simulink model "generic_mcycle"  (Simulink 10.3)
settings: Solver=ode45  StartTime=0.0  StopTime=inf  RelTol=1e-3  EnableMultiTasking=on
libraries: MCycleMaker4SL x1, simulink x1
settings Model: Creator=IPG  LastModifiedBy=IPG  MultithreadedSim=on  ExtModeAutoUpdateStatusClock=off
settings DataIOCC: LimitDataPoints=on  SignalLoggingName=sigsOut
settings OptimizationCC: BooleanDataType=off  InitFltsAndDblsToZero=on
settings DebuggingCC: SaveWithParameterizedLinksMsg=none  SignalResolutionControl=TryResolveAllWithWarning  MultiTaskDSMMsg=warning  MultiTaskCondExecSysMsg=none  SFExecutionAtInitializationDiag=warning
settings HardwareCC: TargetUnknown=on
settings CodeAppCC: MaxIdLength=63
settings GRTTargetCC: TargetFcnLib=ansi_tfl_tmw.mat

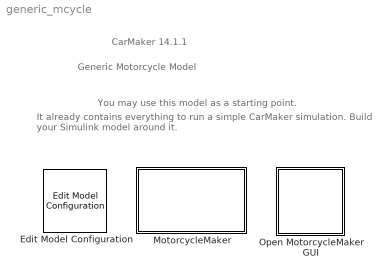
== system generic_mcycle ==
  note: Generic Motorcycle Model
  note: CarMaker 14.1.1
  note: You may use this model as a starting point.
  note: It already contains everything to run a simple CarMaker simulation.
      | Build your Simulink model around it.
  Edit Model Configuration : MCycleMaker4SL/Edit Model Configuration  SFunctionModules=''
  MotorcycleMaker : Subsystem  TreatAsAtomicUnit=on
      mask Display: image(imread('MCycleMakerSys.png'));
  Open MotorcycleMaker GUI : Subsystem  LoadFcn=if ~length(which('cmself')), cmenv; end
      settings: OpenFcn=cmblockmagic('gui_fix_display'); MM_Simulink
      mask Display: image(imread('MCycleMakerGUI.png'));

== system generic_mcycle/MotorcycleMaker ==
  CM_FIRST : Subsystem
  CM_LAST : Subsystem
  DrivMan : Subsystem
  Ground : Ground
  Terminator : Terminator
  Vehicle : Subsystem  TreatAsAtomicUnit=on
  VehicleControl : Subsystem
  wires:
  CM_FIRST/2(Env.Misc) -> DrivMan/2(Env.Misc)
  VehicleControl/2(Vhcl.Model.Source) -> Vehicle/2(Vhcl.Model.Source)
  VehicleControl/7(VhclCtrl.PT) -> Vehicle/7(VhclCtrl.PT)
  VehicleControl/6(VhclCtrl.Brake) -> Vehicle/6(VhclCtrl.Brake)
  VehicleControl/5(Vhcl.Misc) -> Vehicle/5(Vhcl.Misc)
  VehicleControl/4(Vhcl.Wheel.In) -> Vehicle/4(Vhcl.Wheel.In)
  VehicleControl/3(VhclCtrl.Steering) -> Vehicle/3(VhclCtrl.Steering)
  VehicleControl/1(Sync_Out) -> Vehicle/1(Sync_In)
  Vehicle/1(Sync_Out) -> CM_LAST/1(Sync_In)
  Ground/1 -> CM_FIRST/1(Sync_In)
  CM_LAST/1(Sync_Out) -> Terminator/1
  CM_FIRST/1(Sync_Out) -> DrivMan/1(Sync_In)
  DrivMan/1(Sync_Out) -> VehicleControl/1(Sync_In)
  DrivMan/2(DrivMan.Out) -> VehicleControl/2(DrivMan.In)

== system generic_mcycle/Open MotorcycleMaker GUI ==
  S-Function : S-Function  FunctionName=cm_gui  SFunctionDeploymentMode=off  EnableBusSupport=off

== system generic_mcycle/MotorcycleMaker/CM_FIRST ==
  Sync_In : Inport
  BusCreator1 : BusCreator  Inputs=8
  BusCreator2 : BusCreator  Inputs=6
  Demux1 : Demux  Outputs=14
      settings: DisplayOption=none
  Environment : S-Function  FunctionName=MM_Sfun  Parameters='Environment'  SFunctionDeploymentMode=off  EnableBusSupport=off
  IoIn : S-Function  FunctionName=MM_Sfun  Parameters='IoIn'  SFunctionDeploymentMode=off  EnableBusSupport=off
  Terminator : Terminator
  Sync_Out : Outport  VectorParamsAs1DForOutWhenUnconnected=off
  Env.Misc : Outport  Port=2  VectorParamsAs1DForOutWhenUnconnected=off
  wires:
  BusCreator2/1 -> Terminator/1  "IF Environment (in)"
  BusCreator1/1 -> Env.Misc/1
  Demux1/14 -> BusCreator2/6  "Env sRoad"
  Demux1/13 -> BusCreator2/5  "Env PoI_GCS Elev"
  Demux1/12 -> BusCreator2/4  "Env PoI_GCS Lat"
  Demux1/11 -> BusCreator2/3  "Env PoI_GCS Long"
  Demux1/10 -> BusCreator2/2  "Env Time"
  Demux1/9 -> BusCreator2/1  "Env yDay"
  Demux1/8 -> BusCreator1/8  "Env WindVel_tot z"
  Demux1/7 -> BusCreator1/7  "Env WindVel_tot y"
  Demux1/6 -> BusCreator1/6  "Env WindVel_tot x"
  Demux1/5 -> BusCreator1/5  "Env SolarRadiation"
  Demux1/4 -> BusCreator1/4  "Env AirHumidity"
  Demux1/3 -> BusCreator1/3  "Env AirPressure"
  Demux1/2 -> BusCreator1/2  "Env AirDensity"
  Demux1/1 -> BusCreator1/1  "Env Temperature"
  Sync_In/1 -> IoIn/1
  IoIn/1 -> Environment/1
  Environment/1 -> Sync_Out/1
  Environment/2 -> Demux1/1

== system generic_mcycle/MotorcycleMaker/CM_LAST ==
  Sync_In : Inport
  CM_User : S-Function  FunctionName=MM_Sfun  Parameters='CM_User'  SFunctionDeploymentMode=off  EnableBusSupport=off
  IoOut : S-Function  FunctionName=MM_Sfun  Parameters='IoOut'  SFunctionDeploymentMode=off  EnableBusSupport=off
  Sync_Out : Outport  VectorParamsAs1DForOutWhenUnconnected=off
  wires:
  IoOut/1 -> Sync_Out/1
  CM_User/1 -> IoOut/1
  Sync_In/1 -> CM_User/1

== system generic_mcycle/MotorcycleMaker/DrivMan ==
  note: There's rarely a reason to override DrivMan signals.
      | Use the VehicleControl interface for this purpose.
  Sync_In : Inport
  Env.Misc : Inport  Port=2
  BusCreator1 : BusCreator  Inputs=23
  Demux1 : Demux  Outputs=23
      settings: DisplayOption=none
  DrivMan : S-Function  FunctionName=MM_Sfun  Parameters='DrivMan'  SFunctionDeploymentMode=off  EnableBusSupport=off
  Sync_Out : Outport  VectorParamsAs1DForOutWhenUnconnected=off
  DrivMan.Out : Outport  Port=2  VectorParamsAs1DForOutWhenUnconnected=off
  wires:
  Demux1/8 -> BusCreator1/8  "DrivMan SelectorCtrl"
  Demux1/7 -> BusCreator1/7  "DrivMan UserSignal4"
  Demux1/6 -> BusCreator1/6  "DrivMan UserSignal3"
  Demux1/5 -> BusCreator1/5  "DrivMan UserSignal2"
  Demux1/4 -> BusCreator1/4  "DrivMan UserSignal1"
  Demux1/3 -> BusCreator1/3  "DrivMan UserSignal0"
  Demux1/2 -> BusCreator1/2  "DrivMan Key"
  Demux1/1 -> BusCreator1/1  "DrivMan SST"
  DrivMan/1 -> Sync_Out/1
  Sync_In/1 -> DrivMan/1
  Env.Misc/1 -> DrivMan/2
  DrivMan/2 -> Demux1/1
  BusCreator1/1 -> DrivMan.Out/1
  Demux1/9 -> BusCreator1/9  "DrivMan DigitalSelectorCtrl0"
  Demux1/10 -> BusCreator1/10  "DrivMan DigitalSelectorCtrl1"
  Demux1/11 -> BusCreator1/11  "DrivMan DigitalSelectorCtrl2"
  Demux1/23 -> BusCreator1/23  "DrivMan Rider RollAngVel"
  Demux1/22 -> BusCreator1/22  "DrivMan Rider RollAng"
  Demux1/21 -> BusCreator1/21  "DrivMan Steering Trq"
  Demux1/20 -> BusCreator1/20  "DrivMan Steering AngAcc"
  Demux1/19 -> BusCreator1/19  "DrivMan Steering AngVel"
  Demux1/18 -> BusCreator1/18  "DrivMan Steering Ang"
  Demux1/17 -> BusCreator1/17  "DrivMan Gas"
  Demux1/16 -> BusCreator1/16  "DrivMan Clutch"
  Demux1/15 -> BusCreator1/15  "DrivMan BrakePark"
  Demux1/14 -> BusCreator1/14  "DrivMan BrakeLever"
  Demux1/13 -> BusCreator1/13  "DrivMan Brake"
  Demux1/12 -> BusCreator1/12  "DrivMan GearNo"

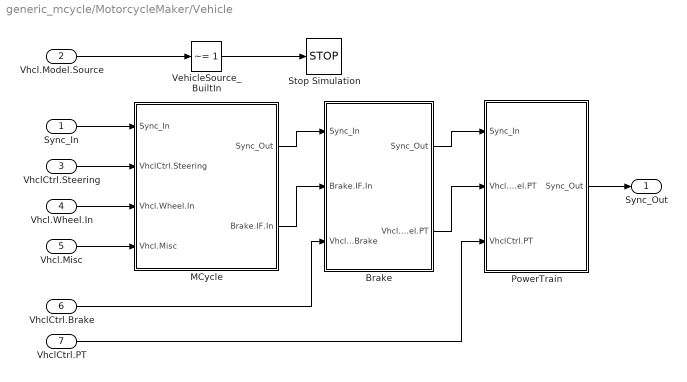
== system generic_mcycle/MotorcycleMaker/Vehicle ==
  Sync_In : Inport
  Vhcl.Model.Source : Inport  Port=2
  VhclCtrl.Steering : Inport  Port=3
  Vhcl.Wheel.In : Inport  Port=4
  Vhcl.Misc : Inport  Port=5
  VhclCtrl.Brake : Inport  Port=6
  VhclCtrl.PT : Inport  Port=7
  Brake : Subsystem
  MCycle : Subsystem
  PowerTrain : Subsystem
  Stop Simulation : Stop
  VehicleSource_BuiltIn : simulink/Logic and Bit Operations/Compare To Constant  relop=~=  const=1  OutDataTypeStr=boolean  ZeroCross=off
  Sync_Out : Outport  VectorParamsAs1DForOutWhenUnconnected=off
  wires:
  Vhcl.Model.Source/1 -> VehicleSource_BuiltIn/1
  Sync_In/1 -> MCycle/1(Sync_In)
  VhclCtrl.Steering/1 -> MCycle/2(VhclCtrl.Steering)
  Vhcl.Wheel.In/1 -> MCycle/3(Vhcl.Wheel.In)
  Vhcl.Misc/1 -> MCycle/4(Vhcl.Misc)
  PowerTrain/1(Sync_Out) -> Sync_Out/1
  VhclCtrl.Brake/1 -> Brake/3(VhclCtrl.Brake)
  MCycle/2(Brake.IF.In) -> Brake/2(Brake.IF.In)
  MCycle/1(Sync_Out) -> Brake/1(Sync_In)
  Brake/1(Sync_Out) -> PowerTrain/1(Sync_In)
  VhclCtrl.PT/1 -> PowerTrain/3(VhclCtrl.PT)
  VehicleSource_BuiltIn/1 -> Stop Simulation/1
  Brake/2(Vhcl.Wheel.PT) -> PowerTrain/2(Vhcl.Wheel.PT)

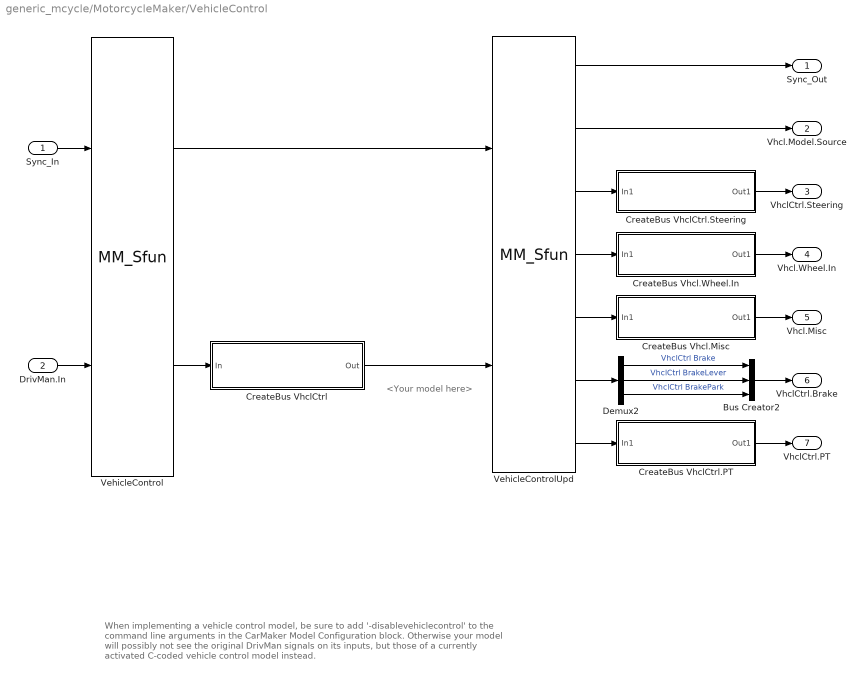
== system generic_mcycle/MotorcycleMaker/VehicleControl ==
  note: When implementing a vehicle control model,
      | be sure to add '-disablevehiclecontrol' to the command line arguments
      | in the CarMaker Model Configuration block.
      | Otherwise your model will possibly not see the original DrivMan signals
      | on its inputs, but those of a currently activated C-coded vehicle control model instead.
  note: <Your model here>
  Sync_In : Inport
  DrivMan.In : Inport  Port=2
  Bus Creator2 : BusCreator  Inputs=3
  CreateBus Vhcl.Misc : Subsystem
  CreateBus Vhcl.Wheel.In : Subsystem
  CreateBus VhclCtrl : Subsystem
  CreateBus VhclCtrl.PT : Subsystem
  CreateBus VhclCtrl.Steering : Subsystem
  Demux2 : Demux  Outputs=3
      settings: DisplayOption=none
  VehicleControl : S-Function  FunctionName=MM_Sfun  Parameters='VehicleControl'  SFunctionDeploymentMode=off  EnableBusSupport=off
  VehicleControlUpd : S-Function  FunctionName=MM_Sfun  Parameters='VehicleControlUpd'  SFunctionDeploymentMode=off  EnableBusSupport=off
  Sync_Out : Outport  VectorParamsAs1DForOutWhenUnconnected=off
  Vhcl.Model.Source : Outport  Port=2  VectorParamsAs1DForOutWhenUnconnected=off
  VhclCtrl.Steering : Outport  Port=3  VectorParamsAs1DForOutWhenUnconnected=off
  Vhcl.Wheel.In : Outport  Port=4  VectorParamsAs1DForOutWhenUnconnected=off
  Vhcl.Misc : Outport  Port=5  VectorParamsAs1DForOutWhenUnconnected=off
  VhclCtrl.Brake : Outport  Port=6  VectorParamsAs1DForOutWhenUnconnected=off
  VhclCtrl.PT : Outport  Port=7  VectorParamsAs1DForOutWhenUnconnected=off
  wires:
  Demux2/1 -> Bus Creator2/1  "VhclCtrl Brake"
  Demux2/2 -> Bus Creator2/2  "VhclCtrl BrakeLever"
  VehicleControlUpd/1 -> Sync_Out/1
  CreateBus VhclCtrl.Steering/1(Out1) -> VhclCtrl.Steering/1
  Bus Creator2/1 -> VhclCtrl.Brake/1
  CreateBus VhclCtrl.PT/1(Out1) -> VhclCtrl.PT/1
  Sync_In/1 -> VehicleControl/1
  VehicleControl/1 -> VehicleControlUpd/1
  DrivMan.In/1 -> VehicleControl/2
  CreateBus Vhcl.Wheel.In/1(Out1) -> Vhcl.Wheel.In/1
  CreateBus Vhcl.Misc/1(Out1) -> Vhcl.Misc/1
  VehicleControlUpd/3 -> CreateBus VhclCtrl.Steering/1(In1)
  VehicleControlUpd/7 -> CreateBus VhclCtrl.PT/1(In1)
  VehicleControlUpd/6 -> Demux2/1
  VehicleControlUpd/5 -> CreateBus Vhcl.Misc/1(In1)
  VehicleControlUpd/4 -> CreateBus Vhcl.Wheel.In/1(In1)
  VehicleControlUpd/2 -> Vhcl.Model.Source/1
  Demux2/3 -> Bus Creator2/3  "VhclCtrl BrakePark"
  VehicleControl/2 -> CreateBus VhclCtrl/1(In)
  CreateBus VhclCtrl/1(Out) -> VehicleControlUpd/2

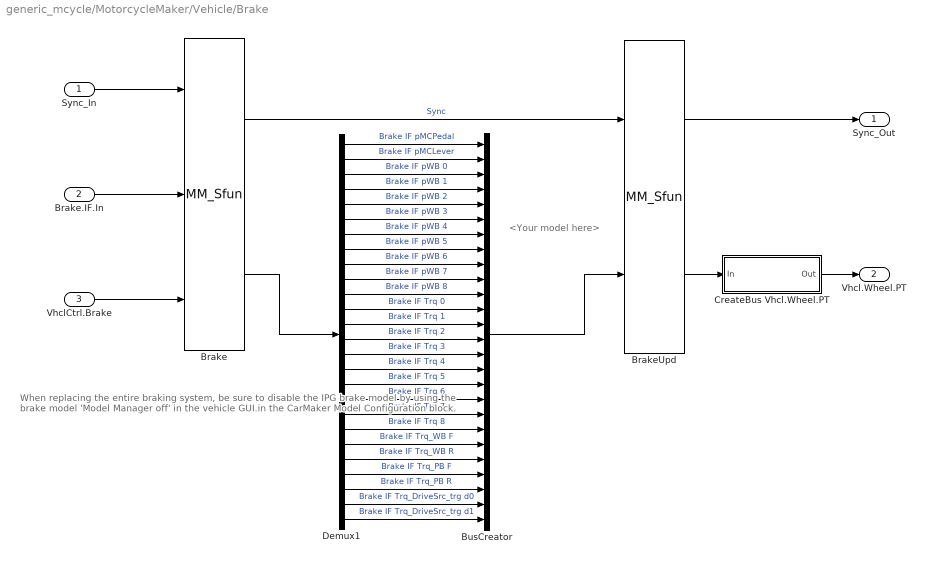
== system generic_mcycle/MotorcycleMaker/Vehicle/Brake ==
  note: When replacing the entire braking system,
      | be sure to disable the IPG brake model by using the brake
      | model 'Model Manager off' in the vehicle GUI.in the CarMaker Model Configuration block.
  note: <Your model here>
  Sync_In : Inport
  Brake.IF.In : Inport  Port=2
  VhclCtrl.Brake : Inport  Port=3
  Brake : S-Function  FunctionName=MM_Sfun  Parameters='Brake'  SFunctionDeploymentMode=off  EnableBusSupport=off
  BrakeUpd : S-Function  FunctionName=MM_Sfun  Parameters='BrakeUpd'  SFunctionDeploymentMode=off  EnableBusSupport=off
  BusCreator : BusCreator  Inputs=26
  CreateBus Vhcl.Wheel.PT : Subsystem
  Demux1 : Demux  Outputs=26
      settings: DisplayOption=none
  Sync_Out : Outport  VectorParamsAs1DForOutWhenUnconnected=off
  Vhcl.Wheel.PT : Outport  Port=2  VectorParamsAs1DForOutWhenUnconnected=off
  wires:
  Demux1/26 -> BusCreator/26  "Brake IF Trq_DriveSrc_trg d1"
  Demux1/25 -> BusCreator/25  "Brake IF Trq_DriveSrc_trg d0"
  Demux1/24 -> BusCreator/24  "Brake IF Trq_PB R"
  Demux1/23 -> BusCreator/23  "Brake IF Trq_PB F"
  Demux1/22 -> BusCreator/22  "Brake IF Trq_WB R"
  Demux1/21 -> BusCreator/21  "Brake IF Trq_WB F"
  Demux1/20 -> BusCreator/20  "Brake IF Trq 8"
  Demux1/19 -> BusCreator/19  "Brake IF Trq 7"
  Demux1/18 -> BusCreator/18  "Brake IF Trq 6"
  Demux1/17 -> BusCreator/17  "Brake IF Trq 5"
  Demux1/16 -> BusCreator/16  "Brake IF Trq 4"
  Demux1/15 -> BusCreator/15  "Brake IF Trq 3"
  Demux1/14 -> BusCreator/14  "Brake IF Trq 2"
  Demux1/13 -> BusCreator/13  "Brake IF Trq 1"
  Demux1/12 -> BusCreator/12  "Brake IF Trq 0"
  Demux1/11 -> BusCreator/11  "Brake IF pWB 8"
  Demux1/10 -> BusCreator/10  "Brake IF pWB 7"
  Demux1/9 -> BusCreator/9  "Brake IF pWB 6"
  Demux1/8 -> BusCreator/8  "Brake IF pWB 5"
  Demux1/7 -> BusCreator/7  "Brake IF pWB 4"
  Demux1/6 -> BusCreator/6  "Brake IF pWB 3"
  Demux1/5 -> BusCreator/5  "Brake IF pWB 2"
  Demux1/4 -> BusCreator/4  "Brake IF pWB 1"
  Demux1/3 -> BusCreator/3  "Brake IF pWB 0"
  Demux1/2 -> BusCreator/2  "Brake IF pMCLever"
  Demux1/1 -> BusCreator/1  "Brake IF pMCPedal"
  Sync_In/1 -> Brake/1
  VhclCtrl.Brake/1 -> Brake/3
  Brake.IF.In/1 -> Brake/2
  Brake/1 -> BrakeUpd/1  "Sync"
  BrakeUpd/1 -> Sync_Out/1
  Brake/2 -> Demux1/1
  BusCreator/1 -> BrakeUpd/2
  BrakeUpd/2 -> CreateBus Vhcl.Wheel.PT/1(In)
  CreateBus Vhcl.Wheel.PT/1(Out) -> Vhcl.Wheel.PT/1

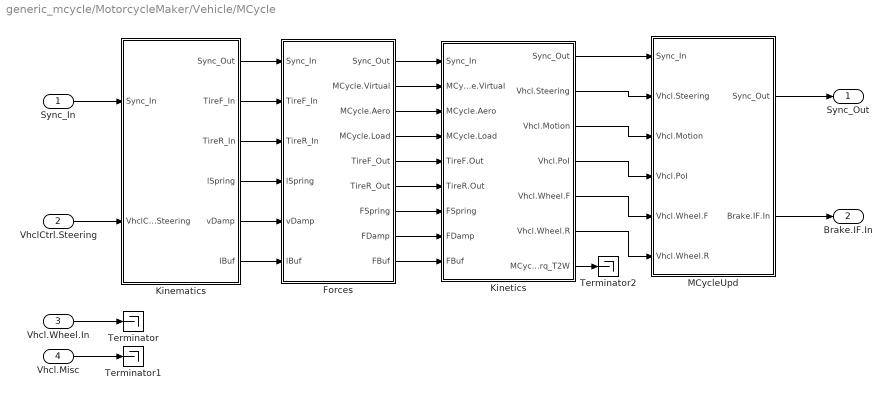
== system generic_mcycle/MotorcycleMaker/Vehicle/MCycle ==
  Sync_In : Inport
  VhclCtrl.Steering : Inport  Port=2
  Vhcl.Wheel.In : Inport  Port=3
  Vhcl.Misc : Inport  Port=4
  Forces : Subsystem
  Kinematics : Subsystem
  Kinetics : Subsystem
  MCycleUpd : Subsystem
  Terminator : Terminator
  Terminator1 : Terminator
  Terminator2 : Terminator
  Sync_Out : Outport  VectorParamsAs1DForOutWhenUnconnected=off
  Brake.IF.In : Outport  Port=2  VectorParamsAs1DForOutWhenUnconnected=off
  wires:
  Vhcl.Wheel.In/1 -> Terminator/1
  Vhcl.Misc/1 -> Terminator1/1
  MCycleUpd/1(Sync_Out) -> Sync_Out/1
  MCycleUpd/2(Brake.IF.In) -> Brake.IF.In/1
  Kinetics/1(Sync_Out) -> MCycleUpd/1(Sync_In)
  Kinetics/2(Vhcl.Steering) -> MCycleUpd/2(Vhcl.Steering)
  Kinetics/3(Vhcl.Motion) -> MCycleUpd/3(Vhcl.Motion)
  Kinetics/4(Vhcl.PoI) -> MCycleUpd/4(Vhcl.PoI)
  Kinetics/5(Vhcl.Wheel.F) -> MCycleUpd/5(Vhcl.Wheel.F)
  Kinetics/6(Vhcl.Wheel.R) -> MCycleUpd/6(Vhcl.Wheel.R)
  Sync_In/1 -> Kinematics/1(Sync_In)
  VhclCtrl.Steering/1 -> Kinematics/2(VhclCtrl.Steering)
  Kinematics/1(Sync_Out) -> Forces/1(Sync_In)
  Kinematics/4(lSpring) -> Forces/4(lSpring)
  Kinematics/5(vDamp) -> Forces/5(vDamp)
  Forces/1(Sync_Out) -> Kinetics/1(Sync_In)
  Forces/2(MCycle.Virtual) -> Kinetics/2(MCycle.Virtual)
  Forces/3(MCycle.Aero) -> Kinetics/3(MCycle.Aero)
  Forces/4(MCycle.Load) -> Kinetics/4(MCycle.Load)
  Forces/7(FSpring) -> Kinetics/7(FSpring)
  Forces/8(FDamp) -> Kinetics/8(FDamp)
  Forces/5(TireF_Out) -> Kinetics/5(TireF.Out)
  Forces/6(TireR_Out) -> Kinetics/6(TireR.Out)
  Kinematics/2(TireF_In) -> Forces/2(TireF_In)
  Kinematics/3(TireR_In) -> Forces/3(TireR_In)
  Kinetics/7(MCycle.Trq_T2W) -> Terminator2/1
  Forces/9(FBuf) -> Kinetics/9(FBuf)
  Kinematics/6(lBuf) -> Forces/6(lBuf)

== system generic_mcycle/MotorcycleMaker/Vehicle/PowerTrain ==
  note: <Your model here>
  note: When replacing the entire powertrain,
      | be sure to disable the IPG powertrain model by using the powertrain
      | model 'Model Manager off' in the vehicle GUI.
  Sync_In : Inport
  Vhcl.Wheel.PT : Inport  Port=2
  VhclCtrl.PT : Inport  Port=3
  BusCreator : BusCreator  Inputs=23
  Demux : Demux  Outputs=23
      settings: DisplayOption=none
  PowerTrain : S-Function  FunctionName=MM_Sfun  Parameters='PowerTrain'  SFunctionDeploymentMode=off  EnableBusSupport=off
  PowerTrainUpd : S-Function  FunctionName=MM_Sfun  Parameters='PowerTrainUpd'  SFunctionDeploymentMode=off  EnableBusSupport=off
  Sync_Out : Outport  VectorParamsAs1DForOutWhenUnconnected=off
  wires:
  Demux/23 -> BusCreator/23  "PT IF WR Trq_BrakeReg_max"
  Demux/22 -> BusCreator/22  "PT IF WR Trq_BrakeReg"
  Demux/21 -> BusCreator/21  "PT IF WR Trq_Supp2WC"
  Demux/20 -> BusCreator/20  "PT IF WR Trq_Drive"
  Demux/19 -> BusCreator/19  "PT IF WR Trq_B2W"
  Demux/18 -> BusCreator/18  "PT IF WR rotv"
  Demux/17 -> BusCreator/17  "PT IF WR rot"
  Demux/16 -> BusCreator/16  "PT IF WF Trq_BrakeReg_max"
  Demux/15 -> BusCreator/15  "PT IF WF Trq_BrakeReg"
  Demux/14 -> BusCreator/14  "PT IF WF Trq_Supp2WC"
  Demux/13 -> BusCreator/13  "PT IF WF Trq_Drive"
  Demux/12 -> BusCreator/12  "PT IF WF Trq_B2W"
  Demux/11 -> BusCreator/11  "PT IF WF rotv"
  Demux/10 -> BusCreator/10  "PT IF WF rot"
  Demux/9 -> BusCreator/9  "PT IF DL_iDiff_mean"
  Demux/8 -> BusCreator/8  "PT IF Trq_Supp2Bdy1 z"
  Demux/7 -> BusCreator/7  "PT IF Trq_Supp2Bdy1 y"
  Demux/6 -> BusCreator/6  "PT IF Trq_Supp2Bdy1 x"
  Demux/5 -> BusCreator/5  "PT IF Engine_rotv"
  Demux/4 -> BusCreator/4  "PT IF GearNo"
  Demux/3 -> BusCreator/3  "PT IF OperationError"
  Demux/2 -> BusCreator/2  "PT IF OperationState"
  Demux/1 -> BusCreator/1  "PT IF Ignition"
  BusCreator/1 -> PowerTrainUpd/2
  PowerTrain/1 -> PowerTrainUpd/1  "Sync"
  PowerTrainUpd/1 -> Sync_Out/1
  Sync_In/1 -> PowerTrain/1
  PowerTrain/2 -> Demux/1
  VhclCtrl.PT/1 -> PowerTrain/3
  Vhcl.Wheel.PT/1 -> PowerTrain/2

== system generic_mcycle/MotorcycleMaker/VehicleControl/CreateBus Vhcl.Misc ==
  In1 : Inport
  BusCreator : BusCreator  Inputs=6
  Demux : Demux  Outputs=6
      settings: DisplayOption=none
  Out1 : Outport  VectorParamsAs1DForOutWhenUnconnected=off
  wires:
  Demux/6 -> BusCreator/6  "Vhcl Wind_vel_0 z"
  Demux/5 -> BusCreator/5  "Vhcl Wind_vel_0 y"
  Demux/4 -> BusCreator/4  "Vhcl Wind_vel_0 x"
  Demux/3 -> BusCreator/3  "Vhcl Trq_DL2Bdy1 z"
  Demux/2 -> BusCreator/2  "Vhcl Trq_DL2Bdy1 y"
  Demux/1 -> BusCreator/1  "Vhcl Trq_DL2Bdy1 x"
  BusCreator/1 -> Out1/1
  In1/1 -> Demux/1

== system generic_mcycle/MotorcycleMaker/VehicleControl/CreateBus Vhcl.Wheel.In ==
  In1 : Inport
  Bus Creator1 : BusCreator  Inputs=6
  Demux1 : Demux  Outputs=6
      settings: DisplayOption=none
  Out1 : Outport  VectorParamsAs1DForOutWhenUnconnected=off
  wires:
  In1/1 -> Demux1/1
  Bus Creator1/1 -> Out1/1
  Demux1/1 -> Bus Creator1/1  "Vhcl Wheel F Trq_B2WC"
  Demux1/2 -> Bus Creator1/2  "Vhcl Wheel F Trq_DL2WC"
  Demux1/3 -> Bus Creator1/3  "Vhcl Wheel F rotv"
  Demux1/4 -> Bus Creator1/4  "Vhcl Wheel R Trq_B2WC"
  Demux1/5 -> Bus Creator1/5  "Vhcl Wheel R Trq_DL2WC"
  Demux1/6 -> Bus Creator1/6  "Vhcl Wheel R rotv"

== system generic_mcycle/MotorcycleMaker/VehicleControl/CreateBus VhclCtrl ==
  In : Inport
  BusCreator : BusCreator  Inputs=32
  Demux : Demux  Outputs=32
      settings: DisplayOption=none
  Out : Outport  VectorParamsAs1DForOutWhenUnconnected=off
  wires:
  BusCreator/1 -> Out/1
  In/1 -> Demux/1
  Demux/1 -> BusCreator/1  "VhclCtrl SST"
  Demux/2 -> BusCreator/2  "VhclCtrl Key"
  Demux/3 -> BusCreator/3  "VhclCtrl UserSignal0"
  Demux/4 -> BusCreator/4  "VhclCtrl UserSignal1"
  Demux/5 -> BusCreator/5  "VhclCtrl UserSignal2"
  Demux/6 -> BusCreator/6  "VhclCtrl UserSignal3"
  Demux/7 -> BusCreator/7  "VhclCtrl UserSignal4"
  Demux/8 -> BusCreator/8  "VhclCtrl GearNo"
  Demux/9 -> BusCreator/9  "VhclCtrl SelectorCtrl"
  Demux/10 -> BusCreator/10  "VhclCtrl Brake"
  Demux/11 -> BusCreator/11  "VhclCtrl BrakeLever"
  Demux/12 -> BusCreator/12  "VhclCtrl BrakePark"
  Demux/13 -> BusCreator/13  "VhclCtrl Clutch"
  Demux/14 -> BusCreator/14  "VhclCtrl Gas"
  Demux/15 -> BusCreator/15  "VhclCtrl Steering Ang"
  Demux/16 -> BusCreator/16  "VhclCtrl Steering AngVel"
  Demux/17 -> BusCreator/17  "VhclCtrl Steering AngAcc"
  Demux/18 -> BusCreator/18  "VhclCtrl Steering Trq"
  Demux/19 -> BusCreator/19  "VhclCtrl Rider RollAng"
  Demux/20 -> BusCreator/20  "VhclCtrl Rider RollAngVel"
  Demux/21 -> BusCreator/21  "VhclCtrl Lights LowBeam"
  Demux/22 -> BusCreator/22  "VhclCtrl Lights HighBeam"
  Demux/23 -> BusCreator/23  "VhclCtrl Lights Daytime"
  Demux/24 -> BusCreator/24  "VhclCtrl Lights ParkL"
  Demux/25 -> BusCreator/25  "VhclCtrl Lights ParkR"
  Demux/26 -> BusCreator/26  "VhclCtrl Lights IndL"
  Demux/27 -> BusCreator/27  "VhclCtrl Lights IndR"
  Demux/28 -> BusCreator/28  "VhclCtrl Lights FogFrontL"
  Demux/29 -> BusCreator/29  "VhclCtrl Lights FogFrontR"
  Demux/30 -> BusCreator/30  "VhclCtrl Lights FogRear"
  Demux/31 -> BusCreator/31  "VhclCtrl Lights Brake"
  Demux/32 -> BusCreator/32  "VhclCtrl Lights Reverse"

== system generic_mcycle/MotorcycleMaker/VehicleControl/CreateBus VhclCtrl.PT ==
  In1 : Inport
  BusCreator : BusCreator  Inputs=12
  Demux : Demux  Outputs=12
      settings: DisplayOption=none
  Out1 : Outport  VectorParamsAs1DForOutWhenUnconnected=off
  wires:
  Demux/12 -> BusCreator/12  "VhclCtrl Brake"
  Demux/11 -> BusCreator/11  "VhclCtrl Gas"
  Demux/10 -> BusCreator/10  "VhclCtrl Clutch"
  Demux/9 -> BusCreator/9  "VhclCtrl SelectorCtrl"
  Demux/8 -> BusCreator/8  "VhclCtrl GearNo"
  Demux/7 -> BusCreator/7  "VhclCtrl UserSignal4"
  Demux/6 -> BusCreator/6  "VhclCtrl UserSignal3"
  Demux/5 -> BusCreator/5  "VhclCtrl UserSignal2"
  Demux/4 -> BusCreator/4  "VhclCtrl UserSignal1"
  Demux/3 -> BusCreator/3  "VhclCtrl UserSignal0"
  Demux/2 -> BusCreator/2  "VhclCtrl Key"
  Demux/1 -> BusCreator/1  "VhclCtrl SST"
  BusCreator/1 -> Out1/1
  In1/1 -> Demux/1

== system generic_mcycle/MotorcycleMaker/VehicleControl/CreateBus VhclCtrl.Steering ==
  In1 : Inport
  BusCreator : BusCreator  Inputs=5
  Demux : Demux  Outputs=5
      settings: DisplayOption=none
  Out1 : Outport  VectorParamsAs1DForOutWhenUnconnected=off
  wires:
  Demux/5 -> BusCreator/5  "VhclCtrl Steering SteerByTrq"
  Demux/4 -> BusCreator/4  "VhclCtrl Steering Trq"
  Demux/3 -> BusCreator/3  "VhclCtrl Steering AngAcc"
  Demux/2 -> BusCreator/2  "VhclCtrl Steering AngVel"
  Demux/1 -> BusCreator/1  "VhclCtrl Steering Ang"
  BusCreator/1 -> Out1/1
  In1/1 -> Demux/1

== system generic_mcycle/MotorcycleMaker/Vehicle/Brake/CreateBus Vhcl.Wheel.PT ==
  In : Inport
  BusCreator : BusCreator  Inputs=8
  Demux : Demux  Outputs=8
      settings: DisplayOption=none
  Out : Outport  VectorParamsAs1DForOutWhenUnconnected=off
  wires:
  Demux/8 -> BusCreator/8  "Vhcl Trq_DriveSrc_trg d1"
  Demux/7 -> BusCreator/7  "Vhcl Trq_DriveSrc_trg d0"
  Demux/6 -> BusCreator/6  "Vhcl Wheel R Trq_T2W"
  Demux/5 -> BusCreator/5  "Vhcl Wheel R Trq_BrakeReg_trg"
  Demux/4 -> BusCreator/4  "Vhcl Wheel R Trq_Brake"
  Demux/3 -> BusCreator/3  "Vhcl Wheel F Trq_T2W"
  Demux/2 -> BusCreator/2  "Vhcl Wheel F Trq_BrakeReg_trg"
  Demux/1 -> BusCreator/1  "Vhcl Wheel F Trq_Brake"
  BusCreator/1 -> Out/1
  In/1 -> Demux/1

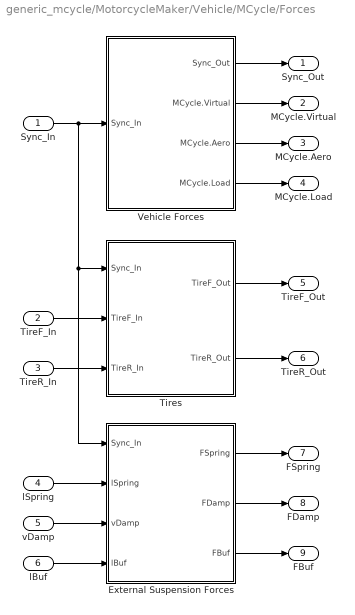
== system generic_mcycle/MotorcycleMaker/Vehicle/MCycle/Forces ==
  Sync_In : Inport
  TireF_In : Inport  Port=2
  TireR_In : Inport  Port=3
  lSpring : Inport  Port=4
  vDamp : Inport  Port=5
  lBuf : Inport  Port=6
  External Suspension Forces : Subsystem
  Tires : Subsystem
  Vehicle Forces : Subsystem
  Sync_Out : Outport  VectorParamsAs1DForOutWhenUnconnected=off
  MCycle.Virtual : Outport  Port=2  VectorParamsAs1DForOutWhenUnconnected=off
  MCycle.Aero : Outport  Port=3  VectorParamsAs1DForOutWhenUnconnected=off
  MCycle.Load : Outport  Port=4  VectorParamsAs1DForOutWhenUnconnected=off
  TireF_Out : Outport  Port=5  VectorParamsAs1DForOutWhenUnconnected=off
  TireR_Out : Outport  Port=6  VectorParamsAs1DForOutWhenUnconnected=off
  FSpring : Outport  Port=7  VectorParamsAs1DForOutWhenUnconnected=off
  FDamp : Outport  Port=8  VectorParamsAs1DForOutWhenUnconnected=off
  FBuf : Outport  Port=9  VectorParamsAs1DForOutWhenUnconnected=off
  wires:
  Sync_In/1 -> Vehicle Forces/1(Sync_In), External Suspension Forces/1(Sync_In), Tires/1(Sync_In)
  Vehicle Forces/1(Sync_Out) -> Sync_Out/1
  Vehicle Forces/2(MCycle.Virtual) -> MCycle.Virtual/1
  Vehicle Forces/3(MCycle.Aero) -> MCycle.Aero/1
  Vehicle Forces/4(MCycle.Load) -> MCycle.Load/1
  lSpring/1 -> External Suspension Forces/2(lSpring)
  External Suspension Forces/2(FDamp) -> FDamp/1
  vDamp/1 -> External Suspension Forces/3(vDamp)
  External Suspension Forces/1(FSpring) -> FSpring/1
  TireF_In/1 -> Tires/2(TireF_In)
  TireR_In/1 -> Tires/3(TireR_In)
  Tires/1(TireF_Out) -> TireF_Out/1
  Tires/2(TireR_Out) -> TireR_Out/1
  lBuf/1 -> External Suspension Forces/4(lBuf)
  External Suspension Forces/3(FBuf) -> FBuf/1

== system generic_mcycle/MotorcycleMaker/Vehicle/MCycle/Kinematics ==
  Sync_In : Inport
  VhclCtrl.Steering : Inport  Port=2
  Kinematics : S-Function  FunctionName=MM_Sfun  Parameters='MCycleKinematics'  SFunctionDeploymentMode=off  EnableBusSupport=off
  Sync_Out : Outport  VectorParamsAs1DForOutWhenUnconnected=off
  TireF_In : Outport  Port=2  VectorParamsAs1DForOutWhenUnconnected=off
  TireR_In : Outport  Port=3  VectorParamsAs1DForOutWhenUnconnected=off
  lSpring : Outport  Port=4  VectorParamsAs1DForOutWhenUnconnected=off
  vDamp : Outport  Port=5  VectorParamsAs1DForOutWhenUnconnected=off
  lBuf : Outport  Port=6  VectorParamsAs1DForOutWhenUnconnected=off
  wires:
  Kinematics/1 -> Sync_Out/1
  VhclCtrl.Steering/1 -> Kinematics/2
  Sync_In/1 -> Kinematics/1
  Kinematics/5 -> vDamp/1
  Kinematics/4 -> lSpring/1
  Kinematics/2 -> TireF_In/1
  Kinematics/3 -> TireR_In/1
  Kinematics/6 -> lBuf/1

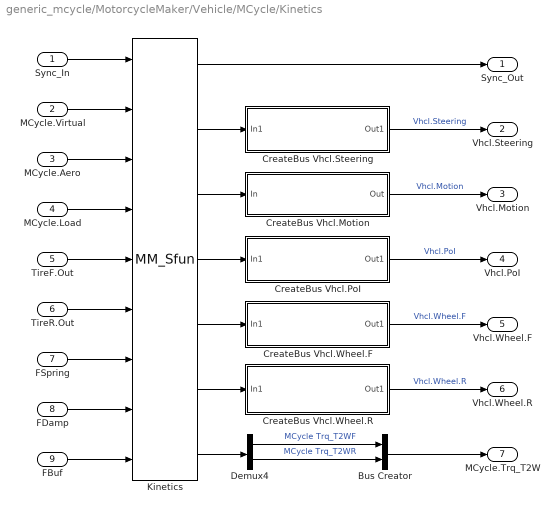
== system generic_mcycle/MotorcycleMaker/Vehicle/MCycle/Kinetics ==
  Sync_In : Inport
  MCycle.Virtual : Inport  Port=2
  MCycle.Aero : Inport  Port=3
  MCycle.Load : Inport  Port=4
  TireF.Out : Inport  Port=5
  TireR.Out : Inport  Port=6
  FSpring : Inport  Port=7
  FDamp : Inport  Port=8
  FBuf : Inport  Port=9
  Bus Creator : BusCreator  Inputs=2
  CreateBus Vhcl.Motion : Subsystem
  CreateBus Vhcl.PoI : Subsystem
  CreateBus Vhcl.Steering : Subsystem
  CreateBus Vhcl.Wheel.F : Subsystem
  CreateBus Vhcl.Wheel.R : Subsystem
  Demux4 : Demux  Outputs=2
      settings: DisplayOption=none
  Kinetics : S-Function  FunctionName=MM_Sfun  Parameters='MCycleKinetics'  SFunctionDeploymentMode=off  EnableBusSupport=off
  Sync_Out : Outport  VectorParamsAs1DForOutWhenUnconnected=off
  Vhcl.Steering : Outport  Port=2  VectorParamsAs1DForOutWhenUnconnected=off
  Vhcl.Motion : Outport  Port=3  VectorParamsAs1DForOutWhenUnconnected=off
  Vhcl.PoI : Outport  Port=4  VectorParamsAs1DForOutWhenUnconnected=off
  Vhcl.Wheel.F : Outport  Port=5  VectorParamsAs1DForOutWhenUnconnected=off
  Vhcl.Wheel.R : Outport  Port=6  VectorParamsAs1DForOutWhenUnconnected=off
  MCycle.Trq_T2W : Outport  Port=7  VectorParamsAs1DForOutWhenUnconnected=off
  wires:
  CreateBus Vhcl.Motion/1(Out) -> Vhcl.Motion/1  "Vhcl.Motion"
  CreateBus Vhcl.PoI/1(Out1) -> Vhcl.PoI/1  "Vhcl.PoI"
  CreateBus Vhcl.Steering/1(Out1) -> Vhcl.Steering/1  "Vhcl.Steering"
  CreateBus Vhcl.Wheel.R/1(Out1) -> Vhcl.Wheel.R/1  "Vhcl.Wheel.R"
  CreateBus Vhcl.Wheel.F/1(Out1) -> Vhcl.Wheel.F/1  "Vhcl.Wheel.F"
  Kinetics/1 -> Sync_Out/1
  Kinetics/2 -> CreateBus Vhcl.Steering/1(In1)
  Kinetics/3 -> CreateBus Vhcl.Motion/1(In)
  Kinetics/4 -> CreateBus Vhcl.PoI/1(In1)
  Kinetics/5 -> CreateBus Vhcl.Wheel.F/1(In1)
  Kinetics/6 -> CreateBus Vhcl.Wheel.R/1(In1)
  Sync_In/1 -> Kinetics/1
  MCycle.Virtual/1 -> Kinetics/2
  MCycle.Aero/1 -> Kinetics/3
  MCycle.Load/1 -> Kinetics/4
  TireF.Out/1 -> Kinetics/5
  TireR.Out/1 -> Kinetics/6
  FSpring/1 -> Kinetics/7
  FDamp/1 -> Kinetics/8
  Demux4/1 -> Bus Creator/1  "MCycle Trq_T2WF"
  Demux4/2 -> Bus Creator/2  "MCycle Trq_T2WR"
  Bus Creator/1 -> MCycle.Trq_T2W/1
  Kinetics/7 -> Demux4/1
  FBuf/1 -> Kinetics/9

== system generic_mcycle/MotorcycleMaker/Vehicle/MCycle/MCycleUpd ==
  Sync_In : Inport
  Vhcl.Steering : Inport  Port=2
  Vhcl.Motion : Inport  Port=3
  Vhcl.PoI : Inport  Port=4
  Vhcl.Wheel.F : Inport  Port=5
  Vhcl.Wheel.R : Inport  Port=6
  CreateBus Brake.IF.In : Subsystem
  MCycleUpd : S-Function  FunctionName=MM_Sfun  Parameters='MCycleUpd'  SFunctionDeploymentMode=off  EnableBusSupport=off
  Sync_Out : Outport  VectorParamsAs1DForOutWhenUnconnected=off
  Brake.IF.In : Outport  Port=2  VectorParamsAs1DForOutWhenUnconnected=off
  wires:
  Sync_In/1 -> MCycleUpd/1
  MCycleUpd/1 -> Sync_Out/1
  CreateBus Brake.IF.In/1(Out1) -> Brake.IF.In/1
  MCycleUpd/2 -> CreateBus Brake.IF.In/1(In1)
  Vhcl.PoI/1 -> MCycleUpd/4
  Vhcl.Motion/1 -> MCycleUpd/3
  Vhcl.Steering/1 -> MCycleUpd/2
  Vhcl.Wheel.F/1 -> MCycleUpd/5
  Vhcl.Wheel.R/1 -> MCycleUpd/6

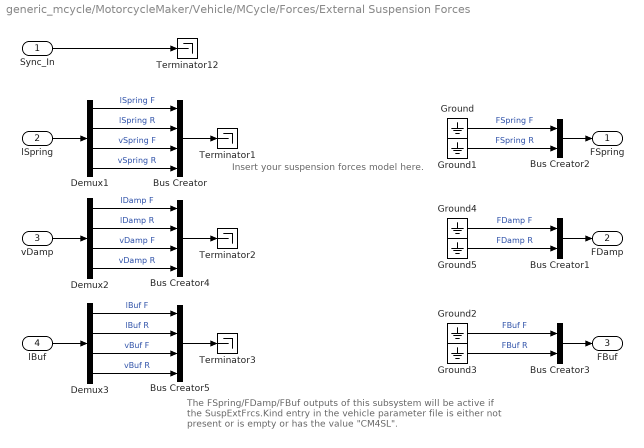
== system generic_mcycle/MotorcycleMaker/Vehicle/MCycle/Forces/External Suspension Forces ==
  note: The FSpring/FDamp/FBuf outputs of this subsystem will be
      | active if the SuspExtFrcs.Kind entry in the vehicle parameter file
      | is either not present or is empty or has the value "CM4SL".
  note: Insert your suspension forces model here.
  Sync_In : Inport
  lSpring : Inport  Port=2
  vDamp : Inport  Port=3
  lBuf : Inport  Port=4
  Bus Creator : BusCreator  Inputs=4
  Bus Creator1 : BusCreator  Inputs=2
  Bus Creator2 : BusCreator  Inputs=2
  Bus Creator3 : BusCreator  Inputs=2
  Bus Creator4 : BusCreator  Inputs=4
  Bus Creator5 : BusCreator  Inputs=4
  Demux1 : Demux
      settings: DisplayOption=none
  Demux2 : Demux
      settings: DisplayOption=none
  Demux3 : Demux
      settings: DisplayOption=none
  Ground{,1..5} (6 alike) : Ground
  Terminator{1..3,12} (4 alike) : Terminator
  FSpring : Outport  VectorParamsAs1DForOutWhenUnconnected=off
  FDamp : Outport  Port=2  VectorParamsAs1DForOutWhenUnconnected=off
  FBuf : Outport  Port=3  VectorParamsAs1DForOutWhenUnconnected=off
  wires:
  Bus Creator5/1 -> Terminator3/1
  Bus Creator4/1 -> Terminator2/1
  Bus Creator/1 -> Terminator1/1
  Demux3/4 -> Bus Creator5/4  "vBuf R"
  Demux3/3 -> Bus Creator5/3  "vBuf F"
  Demux2/4 -> Bus Creator4/4  "vDamp R"
  Demux2/3 -> Bus Creator4/3  "vDamp F"
  Demux1/4 -> Bus Creator/4  "vSpring R"
  Demux1/3 -> Bus Creator/3  "vSpring F"
  Sync_In/1 -> Terminator12/1
  lSpring/1 -> Demux1/1
  vDamp/1 -> Demux2/1
  Demux1/1 -> Bus Creator/1  "lSpring F"
  Demux1/2 -> Bus Creator/2  "lSpring R"
  Demux2/1 -> Bus Creator4/1  "lDamp F"
  Demux2/2 -> Bus Creator4/2  "lDamp R"
  Bus Creator2/1 -> FSpring/1
  Ground4/1 -> Bus Creator1/1  "FDamp F"
  Ground5/1 -> Bus Creator1/2  "FDamp R"
  Bus Creator1/1 -> FDamp/1
  Ground/1 -> Bus Creator2/1  "FSpring F"
  Ground1/1 -> Bus Creator2/2  "FSpring R"
  lBuf/1 -> Demux3/1
  Demux3/1 -> Bus Creator5/1  "lBuf F"
  Demux3/2 -> Bus Creator5/2  "lBuf R"
  Ground2/1 -> Bus Creator3/1  "FBuf F"
  Ground3/1 -> Bus Creator3/2  "FBuf R"
  Bus Creator3/1 -> FBuf/1

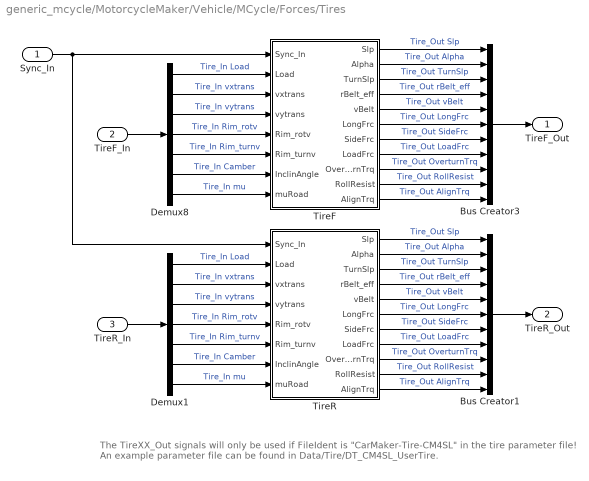
== system generic_mcycle/MotorcycleMaker/Vehicle/MCycle/Forces/Tires ==
  note: The TireXX_Out signals will only be used if FileIdent is "CarMaker-Tire-CM4SL" in the tire parameter file!
      | An example parameter file can be found in Data/Tire/DT_CM4SL_UserTire.
  Sync_In : Inport
  TireF_In : Inport  Port=2
  TireR_In : Inport  Port=3
  Bus Creator1 : BusCreator  Inputs=11
  Bus Creator3 : BusCreator  Inputs=11
  Demux1 : Demux  Outputs=7
      settings: DisplayOption=none
  Demux8 : Demux  Outputs=7
      settings: DisplayOption=none
  TireF : Subsystem
  TireR : Subsystem
  TireF_Out : Outport  VectorParamsAs1DForOutWhenUnconnected=off
  TireR_Out : Outport  Port=2  VectorParamsAs1DForOutWhenUnconnected=off
  wires:
  Sync_In/1 -> TireF/1(Sync_In), TireR/1(Sync_In)
  Bus Creator1/1 -> TireR_Out/1
  Demux1/5 -> TireR/6(Rim_turnv)  "Tire_In Rim_turnv"
  Demux1/4 -> TireR/5(Rim_rotv)  "Tire_In Rim_rotv"
  Demux1/1 -> TireR/2(Load)  "Tire_In Load"
  Demux1/7 -> TireR/8(muRoad)  "Tire_In mu"
  Demux1/6 -> TireR/7(InclinAngle)  "Tire_In Camber"
  Demux1/2 -> TireR/3(vxtrans)  "Tire_In vxtrans"
  Demux1/3 -> TireR/4(vytrans)  "Tire_In vytrans"
  TireR/11(AlignTrq) -> Bus Creator1/11  "Tire_Out AlignTrq"
  TireR/10(RollResist) -> Bus Creator1/10  "Tire_Out RollResist"
  TireR/9(OverturnTrq) -> Bus Creator1/9  "Tire_Out OverturnTrq"
  TireR/8(LoadFrc) -> Bus Creator1/8  "Tire_Out LoadFrc"
  TireR/7(SideFrc) -> Bus Creator1/7  "Tire_Out SideFrc"
  TireR/6(LongFrc) -> Bus Creator1/6  "Tire_Out LongFrc"
  TireR/5(vBelt) -> Bus Creator1/5  "Tire_Out vBelt"
  TireR/4(rBelt_eff) -> Bus Creator1/4  "Tire_Out rBelt_eff"
  TireR/3(TurnSlp) -> Bus Creator1/3  "Tire_Out TurnSlp"
  TireR/1(Slp) -> Bus Creator1/1  "Tire_Out Slp"
  TireR/2(Alpha) -> Bus Creator1/2  "Tire_Out Alpha"
  Demux8/5 -> TireF/6(Rim_turnv)  "Tire_In Rim_turnv"
  Demux8/4 -> TireF/5(Rim_rotv)  "Tire_In Rim_rotv"
  TireF_In/1 -> Demux8/1
  Demux8/1 -> TireF/2(Load)  "Tire_In Load"
  Demux8/7 -> TireF/8(muRoad)  "Tire_In mu"
  Demux8/6 -> TireF/7(InclinAngle)  "Tire_In Camber"
  Demux8/2 -> TireF/3(vxtrans)  "Tire_In vxtrans"
  Demux8/3 -> TireF/4(vytrans)  "Tire_In vytrans"
  TireF/11(AlignTrq) -> Bus Creator3/11  "Tire_Out AlignTrq"
  TireF/10(RollResist) -> Bus Creator3/10  "Tire_Out RollResist"
  TireF/9(OverturnTrq) -> Bus Creator3/9  "Tire_Out OverturnTrq"
  TireF/8(LoadFrc) -> Bus Creator3/8  "Tire_Out LoadFrc"
  TireF/7(SideFrc) -> Bus Creator3/7  "Tire_Out SideFrc"
  TireF/6(LongFrc) -> Bus Creator3/6  "Tire_Out LongFrc"
  TireF/5(vBelt) -> Bus Creator3/5  "Tire_Out vBelt"
  TireF/4(rBelt_eff) -> Bus Creator3/4  "Tire_Out rBelt_eff"
  TireF/3(TurnSlp) -> Bus Creator3/3  "Tire_Out TurnSlp"
  TireF/1(Slp) -> Bus Creator3/1  "Tire_Out Slp"
  TireF/2(Alpha) -> Bus Creator3/2  "Tire_Out Alpha"
  Bus Creator3/1 -> TireF_Out/1
  TireR_In/1 -> Demux1/1

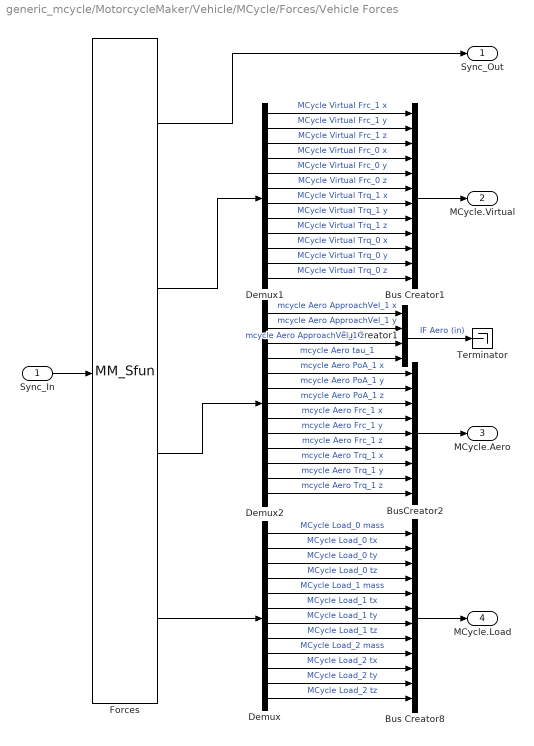
== system generic_mcycle/MotorcycleMaker/Vehicle/MCycle/Forces/Vehicle Forces ==
  Sync_In : Inport
  Bus Creator1 : BusCreator  Inputs=12
  Bus Creator8 : BusCreator  Inputs=12
  BusCreator1 : BusCreator  Inputs=4
  BusCreator2 : BusCreator  Inputs=9
  Demux : Demux  Outputs=12
      settings: DisplayOption=none
  Demux1 : Demux  Outputs=12
      settings: DisplayOption=none
  Demux2 : Demux  Outputs=13
      settings: DisplayOption=none
  Forces : S-Function  FunctionName=MM_Sfun  Parameters='MCycleForces'  SFunctionDeploymentMode=off  EnableBusSupport=off
  Terminator : Terminator
  Sync_Out : Outport  VectorParamsAs1DForOutWhenUnconnected=off
  MCycle.Virtual : Outport  Port=2  VectorParamsAs1DForOutWhenUnconnected=off
  MCycle.Aero : Outport  Port=3  VectorParamsAs1DForOutWhenUnconnected=off
  MCycle.Load : Outport  Port=4  VectorParamsAs1DForOutWhenUnconnected=off
  wires:
  BusCreator1/1 -> Terminator/1  "IF Aero (in)"
  Demux2/13 -> BusCreator2/9  "mcycle Aero Trq_1 z"
  Demux2/12 -> BusCreator2/8  "mcycle Aero Trq_1 y"
  Demux2/11 -> BusCreator2/7  "mcycle Aero Trq_1 x"
  Demux2/10 -> BusCreator2/6  "mcycle Aero Frc_1 z"
  Demux2/9 -> BusCreator2/5  "mcycle Aero Frc_1 y"
  Demux2/8 -> BusCreator2/4  "mcycle Aero Frc_1 x"
  Demux2/7 -> BusCreator2/3  "mcycle Aero PoA_1 z"
  Demux2/6 -> BusCreator2/2  "mcycle Aero PoA_1 y"
  Demux2/5 -> BusCreator2/1  "mcycle Aero PoA_1 x"
  Demux2/4 -> BusCreator1/4  "mcycle Aero tau_1"
  Demux2/3 -> BusCreator1/3  "mcycle Aero ApproachVel_1 z"
  Demux2/2 -> BusCreator1/2  "mcycle Aero ApproachVel_1 y"
  Demux2/1 -> BusCreator1/1  "mcycle Aero ApproachVel_1 x"
  Demux1/12 -> Bus Creator1/12  "MCycle Virtual Trq_0 z"
  Demux1/11 -> Bus Creator1/11  "MCycle Virtual Trq_0 y"
  Demux1/10 -> Bus Creator1/10  "MCycle Virtual Trq_0 x"
  Demux1/9 -> Bus Creator1/9  "MCycle Virtual Trq_1 z"
  Demux1/8 -> Bus Creator1/8  "MCycle Virtual Trq_1 y"
  Demux1/7 -> Bus Creator1/7  "MCycle Virtual Trq_1 x"
  Demux1/6 -> Bus Creator1/6  "MCycle Virtual Frc_0 z"
  Demux1/5 -> Bus Creator1/5  "MCycle Virtual Frc_0 y"
  Demux1/4 -> Bus Creator1/4  "MCycle Virtual Frc_0 x"
  Forces/1 -> Sync_Out/1
  BusCreator2/1 -> MCycle.Aero/1
  Demux1/1 -> Bus Creator1/1  "MCycle Virtual Frc_1 x"
  Demux1/2 -> Bus Creator1/2  "MCycle Virtual Frc_1 y"
  Demux1/3 -> Bus Creator1/3  "MCycle Virtual Frc_1 z"
  Forces/3 -> Demux2/1
  Forces/2 -> Demux1/1
  Bus Creator1/1 -> MCycle.Virtual/1
  Bus Creator8/1 -> MCycle.Load/1
  Demux/1 -> Bus Creator8/1  "MCycle Load_0 mass"
  Demux/2 -> Bus Creator8/2  "MCycle Load_0 tx"
  Demux/3 -> Bus Creator8/3  "MCycle Load_0 ty"
  Demux/4 -> Bus Creator8/4  "MCycle Load_0 tz"
  Demux/5 -> Bus Creator8/5  "MCycle Load_1 mass"
  Demux/6 -> Bus Creator8/6  "MCycle Load_1 tx"
  Demux/7 -> Bus Creator8/7  "MCycle Load_1 ty"
  Demux/8 -> Bus Creator8/8  "MCycle Load_1 tz"
  Demux/9 -> Bus Creator8/9  "MCycle Load_2 mass"
  Demux/10 -> Bus Creator8/10  "MCycle Load_2 tx"
  Demux/11 -> Bus Creator8/11  "MCycle Load_2 ty"
  Demux/12 -> Bus Creator8/12  "MCycle Load_2 tz"
  Forces/4 -> Demux/1
  Sync_In/1 -> Forces/1

== system generic_mcycle/MotorcycleMaker/Vehicle/MCycle/Kinetics/CreateBus Vhcl.Motion ==
  In : Inport
  BusCreator : BusCreator  Inputs=12
  Demux : Demux  Outputs=12
      settings: DisplayOption=none
  Out : Outport  VectorParamsAs1DForOutWhenUnconnected=off
  wires:
  Demux/12 -> BusCreator/12  "Vhcl YawAcc"
  Demux/11 -> BusCreator/11  "Vhcl YawVel"
  Demux/10 -> BusCreator/10  "Vhcl Yaw"
  Demux/9 -> BusCreator/9  "Vhcl PitchAcc"
  Demux/8 -> BusCreator/8  "Vhcl PitchVel"
  Demux/7 -> BusCreator/7  "Vhcl Pitch"
  Demux/6 -> BusCreator/6  "Vhcl RollAcc"
  Demux/5 -> BusCreator/5  "Vhcl RollVel"
  Demux/4 -> BusCreator/4  "Vhcl Roll"
  Demux/3 -> BusCreator/3  "Vhcl sRoad"
  Demux/2 -> BusCreator/2  "Vhcl Distance"
  Demux/1 -> BusCreator/1  "Vhcl v"
  BusCreator/1 -> Out/1
  In/1 -> Demux/1

== system generic_mcycle/MotorcycleMaker/Vehicle/MCycle/Kinetics/CreateBus Vhcl.PoI ==
  In1 : Inport
  Bus Creator3 : BusCreator  Inputs=18
  Demux3 : Demux  Outputs=18
      settings: DisplayOption=none
  Out1 : Outport  VectorParamsAs1DForOutWhenUnconnected=off
  wires:
  Demux3/1 -> Bus Creator3/1  "Vhcl PoI_Pos x"
  Bus Creator3/1 -> Out1/1
  In1/1 -> Demux3/1
  Demux3/2 -> Bus Creator3/2  "Vhcl PoI_Pos y"
  Demux3/3 -> Bus Creator3/3  "Vhcl PoI_Pos z"
  Demux3/4 -> Bus Creator3/4  "Vhcl PoI_Vel x"
  Demux3/5 -> Bus Creator3/5  "Vhcl PoI_Vel y"
  Demux3/6 -> Bus Creator3/6  "Vhcl PoI_Vel z"
  Demux3/7 -> Bus Creator3/7  "Vhcl PoI_Acc x"
  Demux3/8 -> Bus Creator3/8  "Vhcl PoI_Acc y"
  Demux3/9 -> Bus Creator3/9  "Vhcl PoI_Acc z"
  Demux3/10 -> Bus Creator3/10  "Vhcl PoI_Vel_1 x"
  Demux3/11 -> Bus Creator3/11  "Vhcl PoI_Vel_1 y"
  Demux3/12 -> Bus Creator3/12  "Vhcl PoI_Vel_1 z"
  Demux3/13 -> Bus Creator3/13  "Vhcl PoI_Acc_1 x"
  Demux3/14 -> Bus Creator3/14  "Vhcl PoI_Acc_1 y"
  Demux3/15 -> Bus Creator3/15  "Vhcl PoI_Acc_1 z"
  Demux3/16 -> Bus Creator3/16  "Vhcl PoI_GCS Long"
  Demux3/17 -> Bus Creator3/17  "Vhcl PoI_GCS Lat"
  Demux3/18 -> Bus Creator3/18  "Vhcl PoI_GCS Elev"

== system generic_mcycle/MotorcycleMaker/Vehicle/MCycle/Kinetics/CreateBus Vhcl.Steering ==
  In1 : Inport
  Bus Creator3 : BusCreator  Inputs=4
  Demux : Demux
      settings: DisplayOption=none
  Out1 : Outport  VectorParamsAs1DForOutWhenUnconnected=off
  wires:
  In1/1 -> Demux/1
  Demux/4 -> Bus Creator3/4  "Vhcl Steering Trq"
  Demux/2 -> Bus Creator3/2  "Vhcl Steering AngVel"
  Demux/3 -> Bus Creator3/3  "Vhcl Steering AngAcc"
  Demux/1 -> Bus Creator3/1  "Vhcl Steering Ang"
  Bus Creator3/1 -> Out1/1

== system generic_mcycle/MotorcycleMaker/Vehicle/MCycle/Kinetics/CreateBus Vhcl.Wheel.F ==
  In1 : Inport
  Bus Creator3 : BusCreator  Inputs=14
  Demux3 : Demux  Outputs=14
      settings: DisplayOption=none
  Out1 : Outport  VectorParamsAs1DForOutWhenUnconnected=off
  wires:
  Demux3/1 -> Bus Creator3/1  "Vhcl Wheel F t x"
  Bus Creator3/1 -> Out1/1
  In1/1 -> Demux3/1
  Demux3/2 -> Bus Creator3/2  "Vhcl Wheel F t y"
  Demux3/3 -> Bus Creator3/3  "Vhcl Wheel F t z"
  Demux3/4 -> Bus Creator3/4  "Vhcl Wheel F r_zxy x"
  Demux3/5 -> Bus Creator3/5  "Vhcl Wheel F r_zxy y"
  Demux3/6 -> Bus Creator3/6  "Vhcl Wheel F r_zxy z"
  Demux3/7 -> Bus Creator3/7  "Vhcl Wheel F Fx"
  Demux3/8 -> Bus Creator3/8  "Vhcl Wheel F Fy"
  Demux3/9 -> Bus Creator3/9  "Vhcl Wheel F Fz"
  Demux3/10 -> Bus Creator3/10  "Vhcl Wheel F vBelt"
  Demux3/11 -> Bus Creator3/11  "Vhcl Wheel F LongSlip"
  Demux3/12 -> Bus Creator3/12  "Vhcl Wheel F SideSlip"
  Demux3/13 -> Bus Creator3/13  "Vhcl Wheel F Trq_T2W"
  Demux3/14 -> Bus Creator3/14  "Vhcl Wheel F Trq_WhlBearing"

== system generic_mcycle/MotorcycleMaker/Vehicle/MCycle/Kinetics/CreateBus Vhcl.Wheel.R ==
  In1 : Inport
  Bus Creator3 : BusCreator  Inputs=14
  Demux3 : Demux  Outputs=14
      settings: DisplayOption=none
  Out1 : Outport  VectorParamsAs1DForOutWhenUnconnected=off
  wires:
  Demux3/1 -> Bus Creator3/1  "Vhcl Wheel R t x"
  Bus Creator3/1 -> Out1/1
  In1/1 -> Demux3/1
  Demux3/2 -> Bus Creator3/2  "Vhcl Wheel R t y"
  Demux3/3 -> Bus Creator3/3  "Vhcl Wheel R t z"
  Demux3/4 -> Bus Creator3/4  "Vhcl Wheel R r_zxy x"
  Demux3/5 -> Bus Creator3/5  "Vhcl Wheel R r_zxy y"
  Demux3/6 -> Bus Creator3/6  "Vhcl Wheel R r_zxy z"
  Demux3/7 -> Bus Creator3/7  "Vhcl Wheel RFx"
  Demux3/8 -> Bus Creator3/8  "Vhcl Wheel R Fy"
  Demux3/9 -> Bus Creator3/9  "Vhcl Wheel R Fz"
  Demux3/10 -> Bus Creator3/10  "Vhcl Wheel R vBelt"
  Demux3/11 -> Bus Creator3/11  "Vhcl Wheel R LongSlip"
  Demux3/12 -> Bus Creator3/12  "Vhcl Wheel R SideSlip"
  Demux3/14 -> Bus Creator3/14  "Vhcl Wheel R Trq_WhlBearing"
  Demux3/13 -> Bus Creator3/13  "Vhcl Wheel R Trq_T2W"

== system generic_mcycle/MotorcycleMaker/Vehicle/MCycle/MCycleUpd/CreateBus Brake.IF.In ==
  In1 : Inport
  Bus Creator : BusCreator  Inputs=6
  Demux : Demux  Outputs=6
  Out1 : Outport  VectorParamsAs1DForOutWhenUnconnected=off
  wires:
  Demux/1 -> Bus Creator/1  "Brake IF Use_pMCPedalInput"
  Demux/2 -> Bus Creator/2  "Brake IF Use_pMCLeverInput"
  Demux/3 -> Bus Creator/3  "Brake IF pMCPedal_in"
  Demux/4 -> Bus Creator/4  "Brake IF pMCLever_in"
  Demux/5 -> Bus Creator/5  "Brake IF PumpCtrl"
  Demux/6 -> Bus Creator/6  "Brake IF T_env"
  In1/1 -> Demux/1
  Bus Creator/1 -> Out1/1

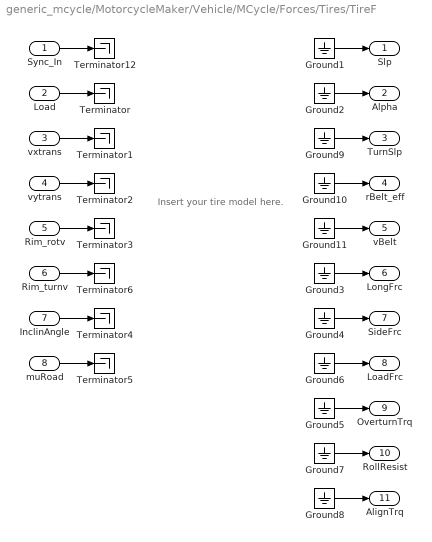
== system generic_mcycle/MotorcycleMaker/Vehicle/MCycle/Forces/Tires/TireF ==
  note: Insert your tire model here.
  Sync_In : Inport
  Load : Inport  Port=2
  vxtrans : Inport  Port=3
  vytrans : Inport  Port=4
  Rim_rotv : Inport  Port=5
  Rim_turnv : Inport  Port=6
  InclinAngle : Inport  Port=7
  muRoad : Inport  Port=8
  Ground{1..11} (11 alike) : Ground
  Terminator{,1..6,12} (8 alike) : Terminator
  Slp : Outport  VectorParamsAs1DForOutWhenUnconnected=off
  Alpha : Outport  Port=2  VectorParamsAs1DForOutWhenUnconnected=off
  TurnSlp : Outport  Port=3  VectorParamsAs1DForOutWhenUnconnected=off
  rBelt_eff : Outport  Port=4  VectorParamsAs1DForOutWhenUnconnected=off
  vBelt : Outport  Port=5  VectorParamsAs1DForOutWhenUnconnected=off
  LongFrc : Outport  Port=6  VectorParamsAs1DForOutWhenUnconnected=off
  SideFrc : Outport  Port=7  VectorParamsAs1DForOutWhenUnconnected=off
  LoadFrc : Outport  Port=8  VectorParamsAs1DForOutWhenUnconnected=off
  OverturnTrq : Outport  Port=9  VectorParamsAs1DForOutWhenUnconnected=off
  RollResist : Outport  Port=10  VectorParamsAs1DForOutWhenUnconnected=off
  AlignTrq : Outport  Port=11  VectorParamsAs1DForOutWhenUnconnected=off
  wires:
  Ground11/1 -> vBelt/1
  Ground10/1 -> rBelt_eff/1
  Ground9/1 -> TurnSlp/1
  Rim_turnv/1 -> Terminator6/1
  Sync_In/1 -> Terminator12/1
  Ground2/1 -> Alpha/1
  Ground3/1 -> LongFrc/1
  Ground4/1 -> SideFrc/1
  Ground5/1 -> OverturnTrq/1
  vxtrans/1 -> Terminator1/1
  vytrans/1 -> Terminator2/1
  Rim_rotv/1 -> Terminator3/1
  InclinAngle/1 -> Terminator4/1
  muRoad/1 -> Terminator5/1
  Load/1 -> Terminator/1
  Ground1/1 -> Slp/1
  Ground6/1 -> LoadFrc/1
  Ground7/1 -> RollResist/1
  Ground8/1 -> AlignTrq/1

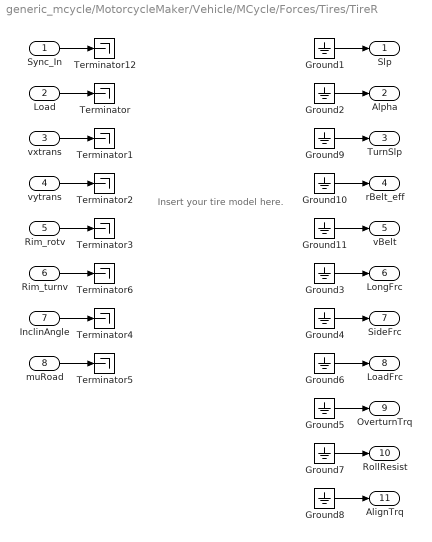
== system generic_mcycle/MotorcycleMaker/Vehicle/MCycle/Forces/Tires/TireR ==
  note: Insert your tire model here.
  Sync_In : Inport
  Load : Inport  Port=2
  vxtrans : Inport  Port=3
  vytrans : Inport  Port=4
  Rim_rotv : Inport  Port=5
  Rim_turnv : Inport  Port=6
  InclinAngle : Inport  Port=7
  muRoad : Inport  Port=8
  Ground{1..11} (11 alike) : Ground
  Terminator{,1..6,12} (8 alike) : Terminator
  Slp : Outport  VectorParamsAs1DForOutWhenUnconnected=off
  Alpha : Outport  Port=2  VectorParamsAs1DForOutWhenUnconnected=off
  TurnSlp : Outport  Port=3  VectorParamsAs1DForOutWhenUnconnected=off
  rBelt_eff : Outport  Port=4  VectorParamsAs1DForOutWhenUnconnected=off
  vBelt : Outport  Port=5  VectorParamsAs1DForOutWhenUnconnected=off
  LongFrc : Outport  Port=6  VectorParamsAs1DForOutWhenUnconnected=off
  SideFrc : Outport  Port=7  VectorParamsAs1DForOutWhenUnconnected=off
  LoadFrc : Outport  Port=8  VectorParamsAs1DForOutWhenUnconnected=off
  OverturnTrq : Outport  Port=9  VectorParamsAs1DForOutWhenUnconnected=off
  RollResist : Outport  Port=10  VectorParamsAs1DForOutWhenUnconnected=off
  AlignTrq : Outport  Port=11  VectorParamsAs1DForOutWhenUnconnected=off
  wires:
  Ground11/1 -> vBelt/1
  Ground10/1 -> rBelt_eff/1
  Ground9/1 -> TurnSlp/1
  Rim_turnv/1 -> Terminator6/1
  Sync_In/1 -> Terminator12/1
  Ground2/1 -> Alpha/1
  Ground3/1 -> LongFrc/1
  Ground4/1 -> SideFrc/1
  Ground5/1 -> OverturnTrq/1
  vxtrans/1 -> Terminator1/1
  vytrans/1 -> Terminator2/1
  Rim_rotv/1 -> Terminator3/1
  InclinAngle/1 -> Terminator4/1
  muRoad/1 -> Terminator5/1
  Load/1 -> Terminator/1
  Ground1/1 -> Slp/1
  Ground6/1 -> LoadFrc/1
  Ground7/1 -> RollResist/1
  Ground8/1 -> AlignTrq/1
